simulink model "kinematicCarComponent"  (R2025b)
settings: Solver=VariableStepAuto  StartTime=0.0  StopTime=10.0  RelTol=1e-3
settings Model: Creator=sprinkle  LastModifiedBy=sprinkle

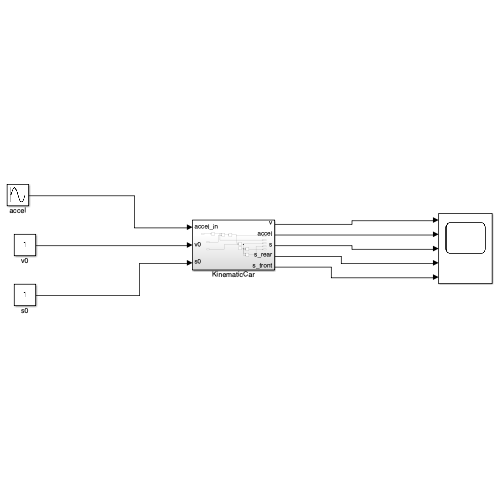
[thumbnail: Simulink's stored preview of the top-level diagram]
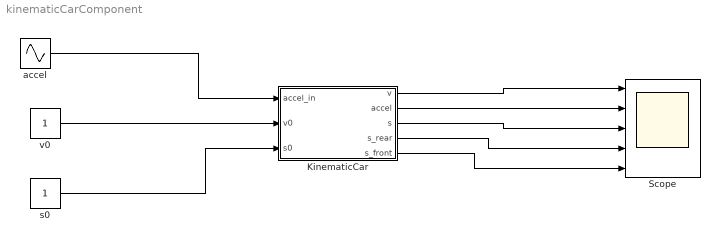
== system kinematicCarComponent ==
  KinematicCar : Subsystem
  Scope : Scope  NumInputPorts=5
      settings: ActiveDisplayYMinimum=-6.4319436824788268  ActiveDisplayYMaximum=22.887493142309445
  accel : Sin  Amplitude=5  SampleTime=0
  s0 : Constant
  v0 : Constant
  wires:
  accel/1 -> KinematicCar/1(accel_in)
  v0/1 -> KinematicCar/2(v0)
  s0/1 -> KinematicCar/3(s0)
  KinematicCar/1(v) -> Scope/1
  KinematicCar/2(accel) -> Scope/2
  KinematicCar/3(s) -> Scope/3
  KinematicCar/4(s_rear) -> Scope/4
  KinematicCar/5(s_front) -> Scope/5

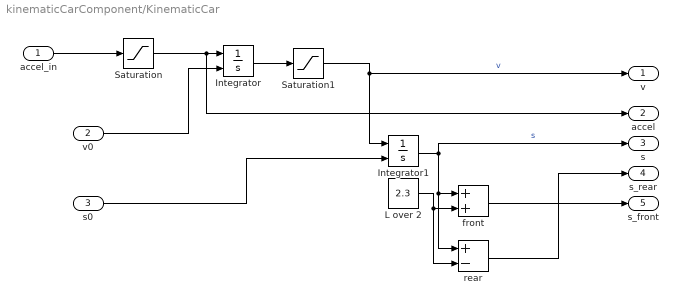
== system kinematicCarComponent/KinematicCar ==
  accel_in : Inport
  v0 : Inport  Port=2
  s0 : Inport  Port=3
  Integrator : Integrator  InitialConditionSource=external
  Integrator1 : Integrator  InitialConditionSource=external
  L over 2 : Constant  Value=2.3
  Saturation : Saturate  UpperLimit=1.5  LowerLimit=-3.5
  Saturation1 : Saturate  UpperLimit=30  LowerLimit=0
  front : Sum
  rear : Sum  Inputs=+-
  v : Outport
  accel : Outport  Port=2
  s : Outport  Port=3
  s_rear : Outport  Port=4
  s_front : Outport  Port=5
  wires:
  front/1 -> s_front/1
  s0/1 -> Integrator1/2
  Saturation/1 -> accel/1, Integrator/1
  v0/1 -> Integrator/2
  L over 2/1 -> rear/2, front/2
  Saturation1/1 -> Integrator1/1, v/1  "v"
  rear/1 -> s_rear/1
  accel_in/1 -> Saturation/1
  Integrator/1 -> Saturation1/1
  Integrator1/1 -> s/1, rear/1, front/1  "s"
